simulink library "INT_AirCtl_DesValCalc"  (R2016b)
settings: Solver=VariableStepAuto  StartTime=0.0  StopTime=10.0  RelTol=1e-3
settings Model: Creator=zhulinfeng  LastModifiedBy=zhulinfeng

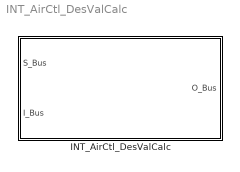
== system INT_AirCtl_DesValCalc ==
  INT_AirCtl_DesValCalc : Subsystem

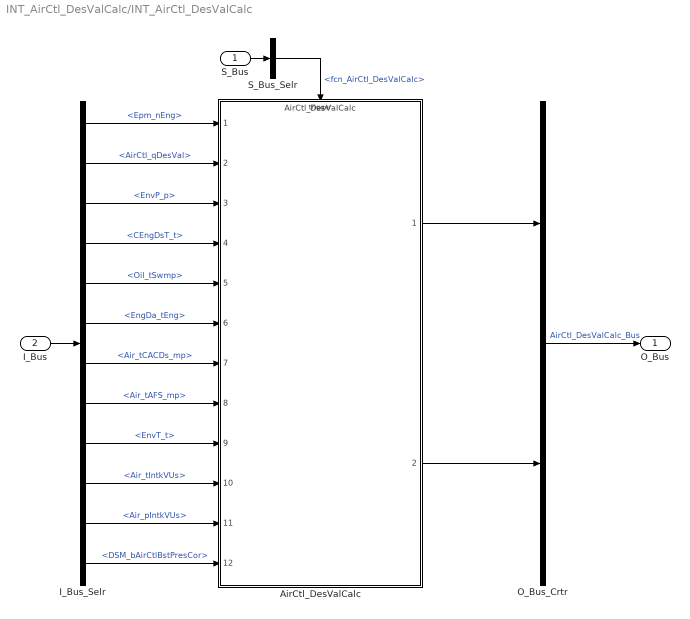
== system INT_AirCtl_DesValCalc/INT_AirCtl_DesValCalc ==
  S_Bus : Inport
  I_Bus : Inport  Port=2
  AirCtl_DesValCalc : ModelReference  ModelNameDialog=AirCtl_DesValCalc  SimulationMode=Normal  ModelReferenceVersion=1.21  TriggerPortName=function  TriggerPortTriggerType=function-call  TriggerPortStatesWhenEnabling=held
  I_Bus_Selr : BusSelector  OutputSignals=Epm_nEng,AirCtl_qDesVal,EnvP_p,CEngDsT_t,Oil_tSwmp,EngDa_tEng,Air_tCACDs_mp,Air_tAFS_mp,EnvT_t,Air_tIntkVUs,Air_pIntkVUs,DSM_bAirCtlBstPresCor
  O_Bus_Crtr : BusCreator  Inputs=2
  S_Bus_Selr : BusSelector  OutputSignals=fcn_AirCtl_DesValCalc
  O_Bus : Outport
  wires:
  S_Bus_Selr/1 -> AirCtl_DesValCalc/Trigger  "<fcn_AirCtl_DesValCalc>"
  S_Bus/1 -> S_Bus_Selr/1
  I_Bus/1 -> I_Bus_Selr/1
  I_Bus_Selr/1 -> AirCtl_DesValCalc/1  "<Epm_nEng>"
  I_Bus_Selr/2 -> AirCtl_DesValCalc/2  "<AirCtl_qDesVal>"
  I_Bus_Selr/3 -> AirCtl_DesValCalc/3  "<EnvP_p>"
  I_Bus_Selr/4 -> AirCtl_DesValCalc/4  "<CEngDsT_t>"
  I_Bus_Selr/5 -> AirCtl_DesValCalc/5  "<Oil_tSwmp>"
  I_Bus_Selr/6 -> AirCtl_DesValCalc/6  "<EngDa_tEng>"
  I_Bus_Selr/7 -> AirCtl_DesValCalc/7  "<Air_tCACDs_mp>"
  I_Bus_Selr/8 -> AirCtl_DesValCalc/8  "<Air_tAFS_mp>"
  I_Bus_Selr/9 -> AirCtl_DesValCalc/9  "<EnvT_t>"
  I_Bus_Selr/10 -> AirCtl_DesValCalc/10  "<Air_tIntkVUs>"
  I_Bus_Selr/11 -> AirCtl_DesValCalc/11  "<Air_pIntkVUs>"
  I_Bus_Selr/12 -> AirCtl_DesValCalc/12  "<DSM_bAirCtlBstPresCor>"
  O_Bus_Crtr/1 -> O_Bus/1  "AirCtl_DesValCalc_Bus"
  AirCtl_DesValCalc/1 -> O_Bus_Crtr/1
  AirCtl_DesValCalc/2 -> O_Bus_Crtr/2
